simulink model "uvms_total"  (Simulink 8.1)
settings: Solver=ode23  StartTime=0.0  StopTime=2  FixedStep=dt  RelTol=1e-4
values from neighbouring files (symbols this model uses):
  DH = struct('a',zeros(n,1),'d',zeros(n,1),'alpha',zeros(n,1))    [init.m]
  dt = 0.01    [run_simulation.m]
undefined symbols (not defined in the file or in its folder): ee_pose_init, ee_pose_quaternion_init, KinematicControlParameters, Kinetics_Parameters, max_zeta, q_init, QLimits, reference_system_matrix_inv, reference_system_zeta_matrix_inv, V_current, vehicle_position_init, vehicle_quaternion_init, VV_States
(part 2 of 2)

== matlab function Kinematic Controller/Event Based Vehicle Control/Calculate VehcileVelocity ==
  data: Measured_States input Bus: measured_states_bus; End_Effector_Com input double; KinematicControlParameters input double; V_vehicle output double size=6; Prev_VV_States input Bus: vehicleVelocityStates_bus; VV_States output Bus: vehicleVelocityStates_bus
function [V_vehicle , VV_States] = getVehicleVelocity(Measured_States,End_Effector_Com, KinematicControlParameters , Prev_VV_States)
%#codegen 
    %% set initial parameters
    VV_States = struct('StatusLinear',0, 'StatusAngular', 0 ,'Circle2EEVec',zeros(3,1), ...
                'linearVehicleVelocity', zeros(6,1), 'angularVehicleVelocity', zeros(6,1) , 'psibe',0, 'V_EE', zeros(6,1), 'VdotP', 0, 'insideWs', 0, 'returnToWi', false);
    
    VV_States.V_EE = End_Effector_Com.velocity;
    VV_States.Circle2EEVec = getVectorCenterOfWsToEE(Measured_States, KinematicControlParameters);  
    VV_States.VdotP = ( Measured_States.Ti.Rbe * VV_States.V_EE(1:3) )' * VV_States.Circle2EEVec;
    VV_States.psibe = getPsibe( Measured_States); 
    
    
    %% check if ee is inside Ws
    p = getEErelativeWs(Measured_States, KinematicControlParameters);
    p = Measured_States.Ti.gbe(1:3,4);
    VV_States.insideWs = checkIfPointIsInsideMesh( KinematicControlParameters.XYZIndices, KinematicControlParameters.XYZPoints, p);
    
    %% Get the status of the vehicle velocity assigner
    StatusLinear = getStatusLinear(Prev_VV_States,VV_States, KinematicControlParameters);
    StatusAngular = getStatusAngular(Prev_VV_States, VV_States, KinematicControlParameters ); 
     
    %% act on the different StatusLinear
    if StatusLinear == 0 
        V_vehicle = zeros(6,1);
        VV_States.returnToWi = false;
    elseif StatusLinear == 1
        V_vehicle = getLinearVelocitySameAsEE( VV_States, Measured_States);
        VV_States.returnToWi = true;
    elseif StatusLinear == 2
        V_vehicle = getReturnToInnerCircleVelocity(VV_States, Measured_States, KinematicControlParameters);
        VV_States.returnToWi = true;
    else
        error('something went wrong in linear states');
    end
    linearVelocity = V_vehicle;
    
    %% act on the different StatusAngular
    if StatusAngular == 0
        V_vehicle = zeros(6,1);
    elseif StatusAngular == 1 
        V_vehicle = getReturnToInnerpsibe(Measured_States, VV_States, KinematicControlParameters);
    else
        error('something went wrong in angular states');
    end
    angularVelocity = V_vehicle;
    
    %% control theta and psi to zero
    R = Measured_States.Ti.R0b;
    phi   = atan2(R(3,2),R(3,3));
    theta = -asin(R(3,1));
    p = - phi;
    q = - theta;
    Kphitheta = KinematicControlParameters.Kphitheta;
    angularVelocity(4:5) = Kphitheta*[p;q] ;
    
    %% set the statuses and the commanded vehicle
    V_vehicle = angularVelocity + linearVelocity;  
    VV_States.StatusLinear = StatusLinear;
    VV_States.StatusAngular = StatusAngular;
    VV_States.linearVehicleVelocity = linearVelocity;
    VV_States.angularVehicleVelocity = angularVelocity;       
end

%------------------------------------------------------------------------------------------------------------------
function V_vehicle = getReturnToInnerpsibe(Measured_States, VV_States, KinematicControlParameters)
    psibe = VV_States.psibe;
    k_ang = KinematicControlParameters.k_ang;
    Vee = VV_States.V_EE;
    omegabe = Vee(4:6);
    Rbe = Measured_States.Ti.Rbe;
    ybe = Measured_States.Ti.pbe(2);
    xbe = Measured_States.Ti.pbe(1);
    % angular velocity of ee around z axis vehicle
    rb0e = [0,0,1] * Rbe * omegabe;
    V_vehicle = [ybe ; -xbe ; 0 ; 0 ; 0 ; 1] * ( rb0e + k_ang * psibe  ) ;    
   
end

%------------------------------------------------------------------------------------------------------------------
function V_vehicle = getLinearVelocitySameAsEE(VV_States, Measured_States)
    Vee = VV_States.V_EE;
    Rbe = Measured_States.Ti.Rbe;
    V_vehicle = zeros(6,1);
    V_vehicle(1:3) = Rbe*Vee(1:3); 
end

%------------------------------------------------------------------------------------------------------------------
function V_vehicle = getAngularSameAsEE(VV_States, Measured_States)
    Vee = VV_States.V_EE;
    omegabe = Vee(4:6);
    Rbe = Measured_States.Ti.Rbe;
    ybe = Measured_States.Ti.pbe(2);
    xbe = Measured_States.Ti.pbe(1);
    % angular velocity of ee around z axis vehicle
    rb0e = [0,0,1] * Rbe * omegabe;
    V_vehicle = [ybe ; -xbe ; 0 ; 0 ; 0 ; 1] * rb0e ;    
end

%------------------------------------------------------------------------------------------------------------------
% get the yaw angle by transforming the forward direction of the end
% effector (z) to the frame of the vehicle, and take the dot product
function psibe  = getPsibe( Measured_States)
    Rbe = Measured_States.Ti.Rbe;
    re = [0,0,1]';
    rb = Rbe * re;
    rb2 = rb(1:2);
    psibe = atan2 ( rb2(2) , rb2(1) );
end



%------------------------------------------------------------------------------------------------------------------
%   create a smooth velocity for the vehicle to make EE return to the inner
%   circle. 
function V_vehicle = getReturnToInnerCircleVelocity(VV_States , Measured_States, KinematicControlParameters)
    Vee = VV_States.V_EE;
    ve = Vee(1:3);
    Rbe = Measured_States.Ti.Rbe;
    k_lin = KinematicControlParameters.k_lin;
    V_vehicle = zeros(6,1);
    V_vehicle(1:3) = Rbe*ve +  k_lin*VV_States.Circle2EEVec./norm( VV_States.Circle2EEVec );

end


%------------------------------------------------------------------------------------------------------------------
%  get the angular status 
%
function StatusAngular = getStatusAngular(Prev_VV_States, VV_States, KinematicControlParameters)
    PrevStatus = Prev_VV_States.StatusAngular;
    psibe = VV_States.psibe;
    prev_psibe = Prev_VV_States.psibe;
    
    if  PrevStatus == 0 && abs(psibe) >= KinematicControlParameters.psis
        StatusAngular = 1;
    elseif abs( psibe ) < KinematicControlParameters.psii
        StatusAngular = 0;
    else
        StatusAngular = PrevStatus;
    end
end

%------------------------------------------------------------------------------------------------------------------
%   the different states are as follows:
%   0 = vehicle steady 
%   1 = outside Ws moving with the end effector
%   2 = moving back to wi 
function StatusLinear = getStatusLinear(Prev_VV_States, VV_States, KinematicControlParameters)
    PrevStatus = Prev_VV_States.StatusLinear;
    VdotP = VV_States.VdotP; 
    Circle2EEVec = VV_States.Circle2EEVec;
    returnToWi = Prev_VV_States.returnToWi;
    
    if norm(Circle2EEVec) < KinematicControlParameters.Wiradius;
        StatusLinear = 0;
    elseif VV_States.insideWs == false && VdotP > 0     
       StatusLinear = 1;
    elseif returnToWi == true
        StatusLinear = 2;
    else
        StatusLinear = PrevStatus;
    end
end

%------------------------------------------------------------------------------------------------------------------
% get the end effectors position relative to the homeposition of Ws
%
function p = getEErelativeWs(Measured_States, KinematicControlParameters)
    pbeInBframe = Measured_States.Ti.gbe(1:3,4);
    p = pbeInBframe - KinematicControlParameters.centerOfWs;
end

%------------------------------------------------------------------------------------------------------------------
% get the vector from the center of ws to ee
function pce = getVectorCenterOfWsToEE(Measured_States, KinematicControlParameters)  
    gbe = Measured_States.Ti.gbe;
    pbe = gbe(1:3,4);
    pbc = KinematicControlParameters.centerOfWs;
    pce = pbe - pbc;    
end

%------------------------------------------------------------------------------------------------------------------
% check if end effector is inside Ws mesh
function isInside = checkIfPointIsInsideMesh (indices, XYZ, point)
    X = XYZ(1,:)';
    Y = XYZ(2,:)';
    Z = XYZ(3,:)';
    idx = indices;
    intersections = 0;
    for i=1:size(indices,1)
        v1 = [ X(idx(i,1)) ; Y(idx(i,1)); Z(idx(i,1)) ]; 
        v2 = [ X(idx(i,2)) ; Y(idx(i,2)); Z(idx(i,2)) ]; 
        v3 = [ X(idx(i,3)) ; Y(idx(i,3)); Z(idx(i,3)) ];
        %intersections = intersections + rayIntersectsTriangle(v1,v2,v3 , point);
        [flag, u, v, t, ray] = rayTriangleIntersection (point,  v1, v2, v3);
        if flag == 1
            intersections = intersections + 1;
        end
    end
    if mod(intersections , 2 ) == 0
       isInside = 0;
    else
       isInside = 1;
    end
end

%------------------------------------------------------------------------------------------------------------------
% Ray/triangle intersection using the algorithm proposed by Möller and Trumbore (1997).
function [flag, u, v, t, ray] = rayTriangleIntersection (o, p0, p1, p2)
    % direction of the ray from the point o
    d = [4,4,4]';
    epsilon = 0.000001;
    e1 = p1-p0;
    e2 = p2-p0;
    q  = cross(d,e2);
    a  = dot(e1,q); % determinant of the matrix M
    if (a>-epsilon && a<epsilon) 
        % the vector is parallel to the plane (the intersection is at infinity)
        [flag, u, v, t,ray] = deal(0,0,0,0,0);
        return;
    end;
    f = 1/a;
    s = o-p0;
    u = f*dot(s,q);
    if (u<0.0)
        % the intersection is outside of the triangle
        [flag, u, v, t, ray] = deal(0,0,0,0,0);
        return;          
    end;
    r = cross(s,e1);
    v = f*dot(d,r);
    if (v<0.0 || u+v>1.0)
        % the intersection is outside of the triangle
        [flag, u, v, t, ray] = deal(0,0,0,0,0);
        return;
    end;
    t = f*dot(e2,r); % verified! 
    if t > epsilon
        flag = 1;
        ray = d;
        return;
    else
        [flag, u, v, t, ray] = deal(0,0,0,0,0);
        return
    end
end

== matlab function Sliding Mode Controller/sliding mode 2/Get error states/MATLAB Function ==
  data: Commanded_States input double; Measured_States input double; Error_States output Bus: error_states_bus
function Error_States = fcn( Commanded_States ,Measured_States)
%#codegen
    Error_States = struct('dzeta_tilde',zeros(12,1), 'zeta_tilde',zeros(12,1),'xi_tilde',zeros(13,1), 'integral_xi_tilde', zeros(13,1),'xi_euler_tilde',zeros(12,1));
    
    p_tilde = Commanded_States.xi(1:3) - Measured_States.xi(1:3);
    Qd = Commanded_States.xi(4:7);
    Q = Measured_States.xi(4:7);
    Q_tilde = getQtilde( Q, Qd);
    q_tilde = Commanded_States.xi(8:13) - Measured_States.xi(8:13);
    
    Error_States.zeta_tilde = Commanded_States.zeta - Measured_States.zeta;
    Error_States.xi_tilde = [p_tilde ; Q_tilde; q_tilde];
end


function Qt = getQtilde(Q, Qd)
    eta = Q(1) ; 
    etad = Qd(1);
    eps = Q(2:4);
    epsd = Qd(2:4);    
    Qt = [...
        eta*etad + eps' * epsd;
        eta*epsd - etad*eps + skew(epsd)*eps
    ];
end

== matlab function Kinematic Controller/Get commanded configuration/Measure States ==
  data: dzeta input double; Commanded_States output Bus: commanded_states_bus; zeta input double; xi input double; q output double
function [Commanded_States , q] = fcn(dzeta, zeta, xi)
%#codegen

Commanded_States.dzeta = dzeta;
Commanded_States.zeta = zeta;
Commanded_States.xi = xi;

Commanded_States.xi_euler = zeros(12,1);
q = xi(8:13);

end

== matlab function Kinematic Controller/Get commanded configuration/zeta2xi/zeta to dot xi ==
  data: zeta input double size=12; dq output double size=6; dp output double size=3; dQ output double size=4; Q input double size=4
function [dq, dp, dQ] = fcn(zeta, Q)                       
    %#codegen
    R0b = Rquat(Q / norm(Q));
    U = getU(Q);
    Ja = [...
            R0b , zeros(3,3) , zeros(3,6);
            zeros(4, 3),  U,    zeros(4,6);
            zeros(6 ,6) , eye(6);
    ];
    
    dXi = Ja * zeta;
    dp = dXi(1:3);
    normalization_feedback = getNormalizationFeedback(Q);   % ensure that the quaternion is unit length
    dQ = dXi(4:7) + normalization_feedback;
    
    dq = dXi(8:13);
end





%----------------------------------------------------------------
%   use normalization feedback according to fossen
%   page 31 to ensure unity of quaternion
function qout = getNormalizationFeedback(qin)
    gamma = 100;
    qout = gamma*0.5*(1-qin'*qin)*qin;
end

%----------------------------------------------------------------
% get the transformation matrix for quaternions
function U = getU(Q)
    eta  = Q(1); eps1 = Q(2); eps2 = Q(3); eps3 = Q(4); 
    U = 0.5*[...
   -eps1 -eps2 -eps3        
    eta  -eps3  eps2
    eps3  eta  -eps1
   -eps2  eps1  eta   ];
end


function R = Rquat(q)
% R = Rquat(q) computes the quaternion rotation matrix R in SO(3)
% for q = [eta eps1 eps2 eps3]
%
% Author:    Thor I. Fossen
% Date:      14th June 2001
% Revisions: 6 October 2001, T I. Fossen - eta as first element in q  
% ________________________________________________________________
%
% MSS GNC is a Matlab toolbox for guidance, navigation and control.
% The toolbox is part of the Marine Systems Simulator (MSS).
%
% Copyright (C) 2008 Thor I. Fossen and Tristan Perez
% 
% This program is free software: you can redistribute it and/or modify
% it under the terms of the GNU General Public License as published by
% the Free Software Foundation, either version 3 of the License, or
% (at your option) any later version.
% 
% This program is distributed in the hope that it will be useful, but
% WITHOUT ANY WARRANTY; without even the implied warranty of
% MERCHANTABILITY or FITNESS FOR A PARTICULAR PURPOSE.  See the 
% GNU General Public License for more details.
% 
% You should have received a copy of the GNU General Public License
% along with this program.  If not, see <http://www.gnu.org/licenses/>.
% 
% E-mail: contact@marinecontrol.org
% URL:    <http://www.marinecontrol.org>

tol = 4*1e-3;
if abs(norm(q)-1)>tol; error('Quaternion not unit. norm(q) must be equal to 1 (in Commanded states)'); end

eta = q(1);
eps = q(2:4);

S = Smtrx(eps);
R = eye(3) + 2*eta*S + 2*S^2;
end

== matlab function Sliding Mode Controller/sliding mode 2/get zetas/get dot y ==
  data: Commanded_States input double; zetas output double size=12; Error_States input double
function zetas  = zetas(Commanded_States , Error_States)
%#codegen
    vd = Commanded_States.zeta(1:3);
    omegad = Commanded_States.zeta(4:6);
    qdd = Commanded_States.zeta(7:12);
    Qd = Commanded_States.xi(4:7);
    x_tilde = Error_States.xi_tilde(1:3);
    eta_tilde = Error_States.xi_tilde(4);
    epsilon_tilde = Error_States.xi_tilde(5:7);
    q_tilde = Error_States.xi_tilde(8:13);
    
    %% vehicle translation
    lambda = 7;
    R = Rquat(Qd);
    zetas1 = vd + lambda* R' * x_tilde;
    
    %% vehicle rotation
    c = 16;
    zetas2 = omegad + 2* c * sgn(eta_tilde)* epsilon_tilde;
    
    %% manipulator
    Kq = diag([1, 1 ,1 ,1 ,1, 1])* 10;
    zetas3 = qdd + Kq*q_tilde;
    
    %% total
    zetas = [zetas1 ; zetas2 ; zetas3];
end

%--------------------------------------------------------
% sgn function returns the sign of the input
function s = sgn(x)
    if x < 0
        s = -1;
    else
        s = 1;
    end
end


%-----------------------------------------------
% get rotation matrix from quaternion
function R = Rquat(Q)
    tol = 2*1e-3;
    if abs(norm(Q)-1)>tol; error('norm(q) must be equal to 1 (In sliding mode controller)'); end
    eta = Q(1);
    eps = Q(2:4);
    S = skew(eps);
    R = eye(3) + 2*eta*S + 2*S^2;
end

== matlab function Sliding Mode Controller/sliding mode 2/Sliding Mode Controller ==
  data: Kinetics_Parameters input Bus: kinetics_bus; tau output double size=12; Measured_States input Bus: measured_states_bus; zetas input double; dzetas input double
function tau  = slidingMode(Kinetics_Parameters, Measured_States, zetas, dzetas)
%#codegen
    zeta = Measured_States.zeta;
    zetar_est = zeta;
    s = zeta - zetas;
    Mest = 0.9*getM(Measured_States, Kinetics_Parameters);
    Cest = 1.2*getC(Measured_States, Kinetics_Parameters, zeta, zetar_est);
    Dest = 1.3*getD(Measured_States, Kinetics_Parameters, zetar_est);
    Nest = 0.75*getN(Measured_States, Kinetics_Parameters);
    Kd=diag([10, 10, 10 ,15, 20, 15, ...
             10, 10, 10, 10, 10, 10])*1;
    Ks=diag([50, 50, 50, 60, 80, 60, ...
             10, 10, 10, 10, 10, 10])*1.5;   
    Xiest = zeros(12,1);
    tau = Mest* dzetas + Cest* zetas + Dest * zetas + Nest + Xiest - Kd* s - Ks*sat( s, 0.9) ;% Ks*sat( s, 0.5);
end

%------------------------------------------------------------------------
% saturation function
function vec = sat (x,epsilon)
    vec=zeros(length(x),1);
    for i=1:length(x)
       if x(i) > epsilon
           vec(i)=1;
       elseif x(i) < -epsilon
           vec(i)=-1;
       else
           vec(i)=x(i)/epsilon;
       end
    end
end


%% --------------------------------------------------------------
%  Functions to gather the vectors   
%%---------------------------------------------------------------

function M = getM(Measured_States, Kinetics_Parameters)
    Mrb = getMrb(Measured_States, Kinetics_Parameters);
    Ma = getMa(Measured_States, Kinetics_Parameters);
    M = (Mrb + Ma);
end


function C = getC (Measured_States,Kinetics_Parameters, zeta ,zetar)
    Crb = getCrb(Measured_States,Kinetics_Parameters, zeta) ;
   	Ca = getCa(Measured_States,Kinetics_Parameters,zetar);
    C = Crb + Ca;
end

%% --------------------------------------------------------------
%  Inertia function   
%%---------------------------------------------------------------
function M = getMrb(Measured_States, Kinetics_Parameters)
%#codegen
%   getMrb Returns the sum of the Rigid body inertia and the added mass:
%   M_rb + M_a
%   
    n=6;
    i=1;
    M = zeros(12,12);
    Inertia = Kinetics_Parameters.Inertia;
    Jgb = [eye(6), zeros(6,6)];                                 % Jacobian from vehicle 
    Ji=Jgb;
    Hi = Kinetics_Parameters.Persistent.Adgici(:,:,i);
    Ii=Hi'*(Inertia(:,:,1))*Hi;                                 % Inertia of vehicle in CO
    M=M+(Ji')*Ii*Ji;
    for i=1:n
        Ji = Measured_States.Ji.Ji(:,:,i);                      % body jacobian
        Hi =Kinetics_Parameters.Persistent.Adgici(:,:,i+1);        % get Transformation matrix of link i
        Ii=Hi'*(Inertia(:,:,i+1) )*Hi;                          % Transform Inertia matrix from CG to CO
        M=M+(Ji')*Ii*Ji;                                        % Add link i's inertia to total inertia
    end
end


%% ------------------------------------------------------
% Persistent Forces   
%%-------------------------------------------------------
function N_p = getN(Measured_States,Kinetics_Parameters)
%#codegen
%   N_p - 12 x 1 vector of generalized forces
%   Persistent_Forces returns the generalized forces due to boyancy and 
%   gravity

    %% init
    n=6;
    N_p=zeros(12,1);
    Jgis = Measured_States.Ji.Ji;
    
    %%  vehicle
    F_bp = getFbp(Measured_States, Kinetics_Parameters,1);      % Get wrench from persistent forces in CO
    Jbb=([eye(6), zeros(6,6)]);                                 % Jacobian from b to b
    N_p = Jbb'*F_bp;                                            % Get contribution to total forces through Jbb
    
    %% robot links
    for i=1:n
        Jgi=Jgis(:,:,i);                                        % Jacobian from b to i
        F_ip = getFip(Measured_States,Kinetics_Parameters, i+1);     % Get wrench in CO
        N_p = N_p + (Jgi')*F_ip;                                % Map to generalized forces and add to total
    end
    N_p = - N_p;                                                % reverse the sign to comply with the sign convention
end
    
    
function F_ip = getFip(Measured_States,Kinetics_Parameters, i)
%#codegen
% function calculating wrench from persistent forces 
% i=b: vehicle
% i>=1: robot arms
    F_ip = zeros(6,1);
    mi = Kinetics_Parameters.Persistent.m(i);
    g = Kinetics_Parameters.Persistent.g;
    rho = Kinetics_Parameters.Persistent.rho;
    nabla = Kinetics_Parameters.Persistent.nabla(i);
    Ri0 = Measured_States.Ti.R0i(:,:,i-1)';
    Adgici = Kinetics_Parameters.Persistent.Adgici(:,:,i);  
    Adgibi = Kinetics_Parameters.Persistent.Adgibi(:,:,i);
    ez=[0;0;1];
    F_ip(:,:) = (Adgici')*[-mi*g*Ri0*ez ;0;0;0]  + (Adgibi')*[rho*nabla*g*Ri0*ez ;0;0;0 ];
end


function F_bp = getFbp(Measured_States,Kinetics_Parameters, i)
%#codegen
% function calculating wrench from persistent forces 
% i=b: vehicle
% i>=1: robot arms
    F_bp = zeros(6,1);
    mi = Kinetics_Parameters.Persistent.m(i);
    g = Kinetics_Parameters.Persistent.g;
    Adgici = Kinetics_Parameters.Persistent.Adgici(:,:,i);  
    Adgibi = Kinetics_Parameters.Persistent.Adgibi(:,:,i);
    rho = Kinetics_Parameters.Persistent.rho;
    nabla = Kinetics_Parameters.Persistent.nabla(i);
    Ri0 = (Measured_States.Ti.R0b)';
    ez=[0;0;1];
    F_bp(:,:) = (Adgici')*[-mi*g*Ri0*ez ; 0;0;0]  + (Adgibi')*[rho*nabla*g*Ri0*ez ; 0;0;0 ];
end


%% ------------------------------------------------------
% Coriolis Matrix   
%%-------------------------------------------------------

function C = getCrb(Measured_States,Kinetics_Parameters, zeta)
%#codegen
%-----------------------------------------------------------------------
%   This function calculates the coriolis according to From and Pettersen
%   (2013).
%-----------------------------------------------------------------------
    n=6;
    C=zeros(12,12);
    Inertia=Kinetics_Parameters.Inertia;
    Jis = Measured_States.Ji.Ji;
    
    % i = b
    Jgb = [eye(6), zeros(6,6)];
    i=1;
    Hi = Kinetics_Parameters.Persistent.Adgici(:,:,i);
    Ii=Hi'*Inertia(:,:,i);
    Wb = getWb(Ii,zeta);
    C = - (Jgb')*Wb*Hi*Jgb;     % time derivative of Jgb = 0  
    
    % i >=1
    for i=1:n
        Hi = Kinetics_Parameters.Persistent.Adgici(:,:,i+1);
        Ii=Hi'*Inertia(:,:,i+1);
        Wi=getWi(Ii,Jis(:,:,i), zeta);
        Jgi_dot=getJgi_dot(Measured_States, zeta,i);
        Jgi = Jis(:,:,i);
        
        C = C + (Jgi')*Ii*Hi*Jgi_dot - (Jgi')*Wi*Hi*Jgi;
    end
end



function Wb = getWb(I , zeta)
%#codegen
% Get the matrix Wi for i=b
% I: Inertia matrix for vehicle
% zeta: generalized velocity
    Wb = zeros(6,6);
    v = zeta(1:3);
    omega = zeta(4:6);
    mI = I(1:3,1:3); % Identity matrix times mass of link b
    Ib = I(4:6,4:6); % Moment of inertia
    mrgb = I(4:6,1:3); % mass times skew symmetric r_g^b
    dKv= mI*v - mrgb*omega;
    dKomega = Ib*omega + mrgb*v;
    
    Wb = [zeros(3,3), skew(dKv) ; skew(dKv), skew(dKomega)];
end

function Wi = getWi(I, Ji,zeta)
%#codegen
% Get matrix Wi for robot links
% I: inertia matrix for link i
% Ji: Jacobian for link i
% zeta: generalized coordinates
    Wi = zeros(6,6);
    V0i = Ji*zeta;
    v = V0i(1:3);
    omega = V0i(4:6);
    mI = I(1:3,1:3); % Identity matrix times mass of link b
    Ib = I(4:6,4:6); % Moment of inertia
    mrgb = I(4:6,1:3); % mass times skew symmetric r_g^b
    dKv= mI*v - mrgb*omega;
    dKomega = Ib*omega + mrgb*v;
    Wi = [zeros(3,3), skew(dKv) ; skew(dKv), skew(dKomega)];
end

function Jgi_dot=getJgi_dot(Measured_States, zeta,i)
%#codegen
% the functions below is related to Jgi_dot
    Jgi_dot = zeros(6,6+6);
    n=6;
    Jgi = Measured_States.Ji.Ji(:,:,i);
    omega = Jgi*zeta;
    Rbi = Measured_States.Ti.Rbi(:,:,i);
    pbi = Measured_States.Ti.pbi(:,i);
    omegaib = getOmegaib(Measured_States,zeta,i);
    dpbi =  getDpbi(Measured_States,zeta,i);
        
    dAdg_inv = [(Rbi')*skew(omegaib) , -(Rbi')*skew(omegaib)*skew(pbi) + (Rbi')*skew(dpbi); ...
                zeros(3,3) , (Rbi')*skew(omegaib) ];
    dJi = zeros(6,6);
    omega0b = zeta(4:6);
    
    % get d/dt(Ji)
    Xii=[0,0,0,0,0,1]';
    for k=2:n
       if k<=i
            dpbk = getDpbi(Measured_States, zeta ,k-1);
            Rbk= Measured_States.Ti.Rbi(:,:,k-1);
            omega0k = [zeros(3,3) , eye(3)]*Measured_States.Ji.Ji(:,:,k-1)*zeta;
            omegabk = omega0k - (Rbk')*omega0b;
            dJi(:,k) = [zeros(3,3), skew(dpbk)*Rbk*skew(omegabk) ...
                ; zeros(3,3) , (Rbk')*skew(omegabk)]*Xii;
       end
    end
    Ji=getji(Measured_States.Ti, i);
    Adg_inv = Measured_States.Ti.Adgbi_inv(:,:,i);
    Jgi_dot = [dAdg_inv, dAdg_inv*Ji + Adg_inv*dJi ];
end

function omegaib = getOmegaib(Measured_States,zeta,i)
%#codegen
% returns angular rate of vehcile wrt frame i noted in vehicle frame
    omegaib = zeros(3,1);
    Rbi = Measured_States.Ti.Rbi(:,:,i);
    Jgi = Measured_States.Ji.Ji(:,:,i);
    omega0b = zeta(4:6);
    omegaib = omega0b - Rbi*[zeros(3,3), eye(3)]*Jgi*zeta;
end

function dpbi = getDpbi( Measured_States, zeta,iter)
%#codegen
% returns time derivative of position vector of from frame b to frame i
    dpbi = zeros(3,1);
    H = [eye(3), zeros(3,3)];
    Rbi=Measured_States.Ti.Rbi(:,:,iter);
    Adgbi_inv = Measured_States.Ti.Adgbi_inv(:,:,iter);
    Ji = getji(Measured_States.Ti,iter);
    qd=zeros(6,1);
    qd(:,:)=zeta(7:12);
    dpbi = Rbi*H*Adgbi_inv*Ji*qd;
end


function mat = getji(Ti,i)
%#codegen
% return matrix Ji (see report)
    n=6;
    mat=zeros(6,6);
    Xii=[0,0,0,0,0,1]';
    mat(:,1)=eye(6)*Xii;
    for j=2:n
        if j<=i
            mat(:,j) = Ti.Adgbi(:,:,j-1)*Xii;
        end
    end
end

function S = skew(v)
%#codegen

  S = [  0   -v(3)  v(2)
       v(3)  0    -v(1)
       -v(2) v(1)   0];
end


%% ------------------------------------------------------
% D matrix 
%%-------------------------------------------------------
function D = getD(Measured_States, Kinetics_Parameters,zetar)
%#codegen
%
% Returns the D matrix in the dynamics equation. The total forces is based
% on mappin the forces in each frame to the total generalized forces
% through the jacoian: tau = J^T*F_i. The forces in frame i is calculated
% from the forces in CG to CO through the transformation matrix: F_co =
% Adgici^T*F_cg
%
    % init
    n=6;
    D=zeros(12,12);                                      % init matrix size
    HydroDynamics = Kinetics_Parameters.HydroDynamics;   % Hydrodynamics parameters
    Jgis = Measured_States.Ji.Ji;                             % Jacobians
    Adgicis = Kinetics_Parameters.Persistent.Adgici;           % Transformation matrix
    
    
    % vehicle
    i=1;
    Jbb=[eye(6), zeros(6)];                               % Jacobian from frame 0 to frame b
    Adgici = Adgicis(:,:,i);                                    % Transformation matrix
    Vcg = Adgici*Jbb*zetar;                                   % velocity in CG mapped from CO
    Dcg =  HydroDynamics.Linear(:,:,i) + ...
           HydroDynamics.Quadratic(:,:,i)*diag(abs(Vcg)); % Wrench in CG
    Di = Adgici'*Dcg;                                        % Wrench in CO mapped from CG    
    D = Jbb'*Di*Jbb;                                      % Add contribution to the total matrix mapped from frame i 
                                                          % to generalized coordinates                                   
    
    % robot links
    for i=1:n
        Jgi = Jgis(:,:,i);                                % Jacobian from frame 0 to frame i 
        Adgici = Adgicis(:,:,i+1);                              % Transformation matrix
        Vcg = Adgici*Jgi*zetar;                               % velocity in CG
        Dcg = HydroDynamics.Linear(:,:,i+1)+... 
          HydroDynamics.Quadratic(:,:,i+1)*diag(abs(Vcg));% Wrench in CG   
        Di = Adgici'*Dcg;                                    % Wrench in CO    
        D = D + Jgi'*Di*Jgi;                              % Add frame i's contribution to D matrix    
    end
end

%% ------------------------------------------------------
% Added Coriolis
%%-------------------------------------------------------
function Ca = getCa(Measured_States,Kinetics_Parameters,zetar)
%%#codegen ..............................................
%
%   This function calculates the added coriolis matrix
%.......................................................
    n=6;
    Ca=zeros(12,12);
    Inertia=Kinetics_Parameters.AddedInertia;
    Jis = Measured_States.Ji.Ji;
    
    % vehicle
    Jgb = [eye(6), zeros(6,6)];
    i=1;
    Hi = Kinetics_Parameters.Persistent.Adgici(:,:,i+1);
    Ii=Hi'*Inertia(:,:,i);
    Wb = getWb(Ii,zetar);
    Ca = - (Jgb')*Wb*Hi*Jgb;     % time derivative of Jgb = 0  
    
    % manipulator links
    for i=1:n
        Hi = Kinetics_Parameters.Persistent.Adgici(:,:,i+1);
        Ii=Hi'*Inertia(:,:,i+1);
        Wi=getWi(Ii,Jis(:,:,i), zetar);
        Jgi_dot=getJgi_dot(Measured_States, zetar,i);
        Jgi = Jis(:,:,i);
        Ca = Ca + (Jgi')*Ii*Hi*Jgi_dot - (Jgi')*Wi*Hi*Jgi;
    end
end

%% ------------------------------------------------------
% Added Mass
%%-------------------------------------------------------
function Ma = getMa(Measured_States,Kinetics_Parameters)
%#codegen ..........................
%
%  returns rest of the the added mass
%  force matrix:
%       Ma*H(xi,zeta)
% ..................................
    n=6;
    i=1;
    
    % get the total Added mass matrix
    Ma = zeros(12,12);
    AddedInertia = Kinetics_Parameters.AddedInertia;
    Jgb = [eye(6), zeros(6,6)];                                 % Jacobian from vehicle 
    Ji=Jgb;
    Hi = Kinetics_Parameters.Persistent.Adgici(:,:,i);
    Ii=Hi'*( AddedInertia(:,:,1))*Hi;                           % Inertia of vehicle in CO
    Ma=Ma+(Ji')*Ii*Ji;
    for i=1:n
        Ji = Measured_States.Ji.Ji(:,:,i);                           % body jacobian
        Hi =Kinetics_Parameters.Persistent.Adgici(:,:,i+1);        % get Transformation matrix of link i
        Ii=Hi'*(AddedInertia(:,:,i+1))*Hi;                      % Transform Inertia matrix from CG to CO
        Ma=Ma+(Ji')*Ii*Ji;                                      % Add link i's inertia to total inertia
    end
 end

== matlab function Kinematic Controller/Reference system/Saturation ==
  data: v_in input double; v_out output double; max_zeta input double
function v_out = fcn(v_in, max_zeta)
%#codegen
    
    v_out = zeros(6,1);
    for i=1:6
       if abs(v_in(i) >= max_zeta(i))
          v_out(i) =  sign(v_in(i)) * max_zeta(i);
       else
           v_out(i) = v_in(i);
       end
    end
end

== matlab function Path generator/End Effector2/MATLAB Function1 ==
  data: velocity input double; End_Effector_Com output Bus: endEffector_com_bus; pose input double
function End_Effector_Com = fcn(velocity,pose)
%#codegen
    End_Effector_Com = struct('velocity', zeros(6,1), 'pose',zeros(7,1));
    End_Effector_Com.pose = pose;
    End_Effector_Com.velocity = velocity;
end

== matlab function Path generator/End Effector2/twist2pose_euler/body2eulervel ==
  data: ee_velocity_twist input double size=6; ee_rates output double size=6; euler_angles_ee input double size=3
function ee_rates = fcn(ee_velocity_twist, euler_angles_ee)                       
    %#codegen
       
    phi=euler_angles_ee(1);
    theta=euler_angles_ee(2);
    psi=euler_angles_ee(3);
    
    
    cphi = cos(phi);
    sphi = sin(phi);
    cth  = cos(theta);
    sth  = sin(theta);
 
    J1 = Rzyx(phi,theta,psi);
 
    if cth==0, error('J2 is singular for theta = +-90 degrees'); end
 
    J2 = [...
      1  sphi*sth/cth  cphi*sth/cth;
      0  cphi          -sphi;
      0  sphi/cth      cphi/cth ];
 
    J = [ J1  zeros(3,3);
      zeros(3,3) J2 ];
        
    ee_rates = zeros(6,1);
    ee_rates=J*ee_velocity_twist;
end



function R = Rzyx(phi,theta,psi)
    cphi = cos(phi);
    sphi = sin(phi);
    cth  = cos(theta);
    sth  = sin(theta);
    cpsi = cos(psi);
    spsi = sin(psi);

    R = [...
       cpsi*cth  -spsi*cphi+cpsi*sth*sphi  spsi*sphi+cpsi*cphi*sth
       spsi*cth  cpsi*cphi+sphi*sth*spsi   -cpsi*sphi+sth*spsi*cphi
       -sth      cth*sphi                  cth*cphi ];
end

== matlab function Path generator/End Effector2/twist2pose_quaternions/MATLAB Function ==
  data: pose output double; quaternion output double; poseIn input double
function [pose, quaternion] = fcn(poseIn)
%#codegen
    pose = poseIn;
    quaternion = poseIn(4:7);
end

== matlab function Path generator/End Effector2/twist2pose_quaternions/body2quat ==
  data: ee_velocity_twist input double size=6; ee_rates output double; quat input double size=4
function ee_rates = fcn(ee_velocity_twist, quat)                       
    %#codegen
    
    eta  = quat(1); 
    eps1 = quat(2); 
    eps2 = quat(3); 
    eps3 = quat(4); 
    
    
    normalization_feedback = getNormalizationFeedback(quat);
    
    v = ee_velocity_twist(1:3);
    omega = ee_velocity_twist(4:6);
    
    R = Rquat(quat);

    T = 0.5*[...
    -eps1 -eps2 -eps3        
    eta  -eps3  eps2
    eps3  eta  -eps1
    -eps2  eps1  eta   ];

    pdot = R*v;
    qdot = T*omega + normalization_feedback;
    
    ee_rates = zeros(7,1);
    ee_rates(:) = [ pdot ; qdot];
    
    
end



function R = Rquat(q)
%#codegen
eta = q(1);
eps = q(2:4);
S = skew(eps);
R = eye(3) + 2*eta*S + 2*S^2;

end


function S = skew(v)
%#codegen
    S = [  0   -v(3)  v(2)
       v(3)  0    -v(1)
       -v(2) v(1)   0];
end


%----------------------------------------------------------------
%   use normalization feedback according to fossen
%   page 31
function qout = getNormalizationFeedback(qin)
%#codegen
    qout = zeros(4,1);
    gamma = 100;
    qout = gamma*0.5*(1-qin'*qin)*qin;

end

== matlab function Path generator/EE velocity in frame 0 to EE velocity in frame e ==
  data: pose input double; V0 input double; Vb output double
function Vb= fcn(pose, V0)
%#codegen
    euler_angles_ee = pose(4:6);
    phi=euler_angles_ee(1);
    theta=euler_angles_ee(2);
    psi=euler_angles_ee(3);
        
    cphi = cos(phi);
    sphi = sin(phi);
    cth  = cos(theta);
    sth  = sin(theta);
    R = Rzyx(phi,theta,psi);
    if cth==0, error('J2 is singular for theta = +-90 degrees'); end
    T_inv = [...
        1,0,-sth;
        0,cphi,cth*sphi;
        0,-sphi,cth*cphi
    ];
    J = [ R' , zeros(3,3);
          zeros(3,3), T_inv ];
    Vb=J*V0;
end



function R = Rzyx(phi,theta,psi)
    cphi = cos(phi);
    sphi = sin(phi);
    cth  = cos(theta);
    sth  = sin(theta);
    cpsi = cos(psi);
    spsi = sin(psi);

    R = [...
       cpsi*cth  -spsi*cphi+cpsi*sth*sphi  spsi*sphi+cpsi*cphi*sth
       spsi*cth  cpsi*cphi+sphi*sth*spsi   -cpsi*sphi+sth*spsi*cphi
       -sth      cth*sphi                  cth*cphi ];
end

== matlab function UVMS/Kinetics/Measure states/End Effector Motion ==
  data: Kinematics input double; zeta input double; Vee output double
function Vee = fcn(Kinematics,  zeta)
%#codegen
    Je = Kinematics.Ji.Je;
    Vee = Je*zeta;
end

== matlab function UVMS/Kinetics/Measure states/twist2pose_quaternions/MATLAB Function ==
  data: pose output double; quaternion output double; poseIn input double
function [pose, quaternion] = fcn(poseIn)
%#codegen
    pose = poseIn;
    quaternion = poseIn(4:7);
end

== matlab function UVMS/Kinetics/Measure states/twist2pose_quaternions/body2quat ==
  data: ee_velocity_twist input double size=6; ee_rates output double; quat input double
function ee_rates = fcn(ee_velocity_twist, quat)                       
    %#codegen
    
    eta  = quat(1); 
    eps1 = quat(2); 
    eps2 = quat(3); 
    eps3 = quat(4); 
    
    
    normalization_feedback = getNormalizationFeedback(quat);
    
    v = ee_velocity_twist(1:3);
    omega = ee_velocity_twist(4:6);
    
    
    R = Rquat(quat);

    T = 0.5*[...
    -eps1 -eps2 -eps3        
    eta  -eps3  eps2
    eps3  eta  -eps1
    -eps2  eps1  eta   ];

    pdot = R*v;
    qdot = T*omega + normalization_feedback;
    
    ee_rates = zeros(7,1);
    ee_rates(:) = [pdot;    qdot];
    
end



function R = Rquat(q)
%#codegen
eta = q(1);
eps = q(2:4);
S = skew(eps);
R = eye(3) + 2*eta*S + 2*S^2;

end


function S = skew(v)
%#codegen
    S = [  0   -v(3)  v(2)
       v(3)  0    -v(1)
       -v(2) v(1)   0];
end


%----------------------------------------------------------------
%   use normalization feedback according to fossen
%   page 31
%
function qout = getNormalizationFeedback(qin)
%#codegen
    qout = zeros(4,1);
    gamma = 100;
    qout = gamma*0.5*(1-qin'*qin)*qin;

end
